simulink model "battery2"  (R2023b)
settings: Solver=VariableStepAuto  StartTime=0.0  StopTime=inf  RelTol=1e-3
undefined symbols (not defined in the file): AH, R0
libraries: BatteryEstimators x1
settings Model: Creator=chris  LastModifiedBy=chris

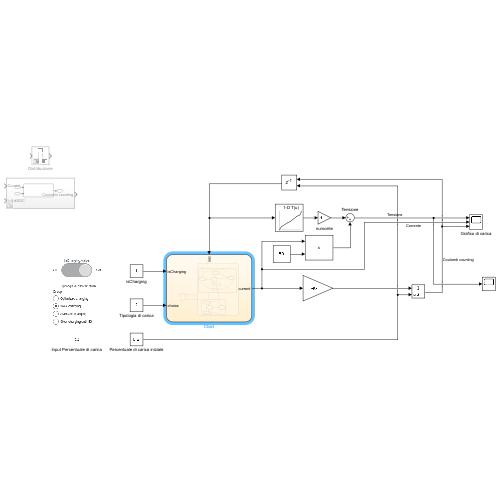
[thumbnail: Simulink's stored preview of the top-level diagram]
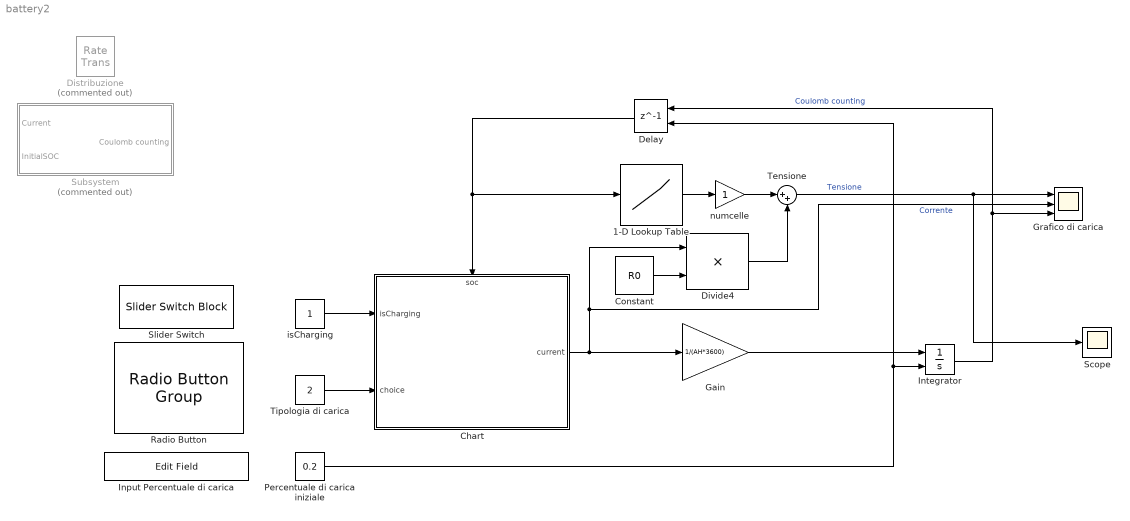
== system battery2 ==
  1-D Lookup Table : Lookup_n-D  NumberOfTableDimensions=1  BreakpointsForDimension1=[0, .1, .38,.511,.8,.92, 1]  Table=[3.28, 3.45, 3.63, 3.69,3.95,4.01,4.2]  InternalRulePriority=Speed  RndMeth=Simplest
  Chart : Stateflow chart  TreatAsAtomicUnit=on
      settings: PortSchema="{\"entries\":[{\"content\":{\"sides\":[{\"content\":{\"connectorIds\":[\"In1\",\"In3\"]},\"type\":\"ConnectorPlacement.EquallySpacedRectSide\",\"uuid\":\"a6672bef-1ba0-496b-9c5e-64820f88021e\"},{\"content\":{\"connectorIds\":[\"Out1\"],\"side\":\"RIGHT\"},\"type\":\"ConnectorPlacement.EquallySpacedRectSide\",\"uuid\":\"9e4eb33c-d745-4260-a0dc-36479670b9dc\"},{\"content\":{\"connectorIds\":[\"In2\"],\"side\":\"TOP\"},\"type\":\"ConnectorPlacement.EquallySpacedRectSide\",\"uuid\":\"ece41cf9-1d3b-45f4-8ae6-354b3a498270\"},{\"content\":{\"side\":\"BOTTOM\"},\"type\":\"ConnectorPlacement.EquallySpacedRectSide\",\"uuid\":\"edd66967-5ff2-47ba-bdfe-f7b79a318669\"}]},\"type\":\"ConnectorPlacement.EquallySpacedConnector\",\"uuid\":\"4cccf6ba-1acf-421a-acb7-d2646cbad516\"}],\"packageUris\":[\"http://schema.mathworks.com/mf0/Connector/R2020b\"],\"version\":\"1.0\"}"
  Constant : Constant  Value=R0
  Delay : Delay  DelayLength=1  InitialConditionSource=Input port
      settings: InputPortMap=u0,p4
  Distribuzione : RateTransition  Commented=on  InitialCondition=0.1
  Divide4 : Product  Inputs=**
  Gain : Gain  Gain=1/(AH*3600)
  Grafico di carica : Scope  NumInputPorts=3
  Input Percentuale di carica : EditField  LabelPosition=Hide  ShowInitialText=on  Alignment=Center
  Integrator : Integrator  InitialConditionSource=external
  Percentuale di carica iniziale : Constant  Value=0.2
  Radio Button : RadioButtonGroup  SelectedLabel=Slow charging  ButtonGroupName=Group
      settings: Values={{'Optimized charging', 'Slow charging', 'Standard charging', 'Slow charging until 80'}, [1 2 3 4]}
  Scope : Scope
  Slider Switch : SliderSwitchBlock
      settings: Values={{'Off', 'On'}, [0 1]}
  Subsystem : Subsystem  Commented=on
  Tensione : Sum  Inputs=|++
  Tipologia di carica : Constant  Value=2
  isCharging : Constant
  numcelle : Gain
  wires:
  Constant/1 -> Divide4/2
  Divide4/1 -> Tensione/2
  Tipologia di carica/1 -> Chart/3(choice)
  Tensione/1 -> Scope/1, Grafico di carica/1  "Tensione"
  Gain/1 -> Integrator/1
  Delay/1 -> 1-D Lookup Table/1, Chart/2(soc)
  1-D Lookup Table/1 -> numcelle/1
  Chart/1(current) -> Grafico di carica/2, Divide4/1, Gain/1  "Corrente"
  isCharging/1 -> Chart/1(isCharging)
  numcelle/1 -> Tensione/1
  Integrator/1 -> Grafico di carica/3, Delay/1  "Coulomb counting"
  Percentuale di carica iniziale/1 -> Delay/2, Integrator/2

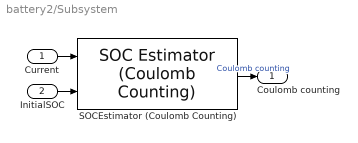
== system battery2/Subsystem ==
  Current : Inport
  InitialSOC : Inport  Port=2
  SOCEstimator (Coulomb Counting) : BatteryEstimators/SOC Estimator (Coulomb Counting)  CurrentInputPartition=off  AH=3  Ts=2
      settings: LibrarySourceBlock=|
      | batt_sl_lib/Estimators/SOC Estimator
      | (Coulomb Counting)
  Coulomb counting : Outport
  wires:
  SOCEstimator (Coulomb Counting)/1 -> Coulomb counting/1  "Coulomb counting"
  InitialSOC/1 -> SOCEstimator (Coulomb Counting)/2
  Current/1 -> SOCEstimator (Coulomb Counting)/1

== stateflow chart battery2/Chart ==
  settings: updateMethod=CONTINUOUS  sampleTime=1
  state BatteryOn1
    state Charging
      state FastCharge
        en: current = 3
      state SlowCharge
        en: current = 1
      state gest1
      state regular
        en: current = 1.5
      state slowChargeuntil80
        en: current = 1
      state idle
        en: current = 0
      regular -> SlowCharge [order 2] : [soc >= 0.5]
      FastCharge -> SlowCharge : [soc >= 0.7]
      gest1 -> FastCharge [order 1] : [choice == 1]
      (default) -> gest1
      gest1 -> SlowCharge [order 2] : [choice ==2]
      gest1 -> regular [order 3] : [choice == 3]
      SlowCharge -> idle : [soc>=0.98]
      regular -> idle [order 1] : [soc>=0.98]
      gest1 -> slowChargeuntil80 [order 4] : [choice == 4]
      slowChargeuntil80 -> idle : [soc >= 0.78]
    note: corrente negativa sarebbe consumo di corrente
    state Discharging
      state PerformanceMode
        en: current = - 3
      state normalmode
        en: current = - 1.5
      state Manager
      state BatterySaverMode
        en: current = - 1
      PerformanceMode -> normalmode : [soc < 0.5]
      Manager -> PerformanceMode [order 2] : [soc >= 0.8]
      Manager -> normalmode [order 1] : [soc > 0.2 & soc < 0.8]
      (default) -> Manager
      normalmode -> BatterySaverMode : [soc < 0.2]
      Manager -> BatterySaverMode [order 3] : [soc <= 0.2 ]
    (default) -> Charging
    Charging -> Discharging : [isCharging == 0]
    Discharging -> Charging : [isCharging == 1 ]
  state Batteryoff
    en: current = 0
  (default) -> BatteryOn1
  BatteryOn1 -> Batteryoff : [soc<=0.01 && isCharging == 0]
  Batteryoff -> BatteryOn1 : [isCharging == 1]
  data: isCharging input; current output =0; soc input; choice input
  data current settings: updateMethod=SF_CONTINUOUS_TIME_DATA
